simulink model "Robot2dof_control_Friction_RBFNN"  (Simulink 8.5)
settings: Solver=ode45  StartTime=0.0  StopTime=20  RelTol=1e-3
values from neighbouring files (symbols this model uses):
  l1 = 1    [Inv_Kinematic.m]    (also in Parameters.m)
  l2 = 0.5    [Inv_Kinematic.m]    (also in Parameters.m)
  m1 = 2    [Parameters.m]
  m2 = 1    [Parameters.m]
libraries: mblibv1 x13
(part 2 of 2)

== matlab function Computed Torque Controller/Computed Torque/Computed torque controller ==
  data: q1 input double; Torque1 output double; Torque2 output double; q2 input double; q1_dot input double; q2_dot input double; qd1 input double; qd2 input double; qd1_dot input double; qd2_dot input double; qd1_dotdot input double; qd2_dotdot input double
function [Torque1,Torque2] = ComputedTorqueController(q1,q2,q1_dot,q2_dot,qd1,qd2,qd1_dot,qd2_dot,qd1_dotdot,qd2_dotdot)
%% Adjust the inputs to apply the formulas
%   q2 is initially the complement angle of link 2 to link 1.
%   In order to apply the formulas, we need to determine the angle 
%   between link 2 and the x-axis to apply the dynamic model.
%   The same things go to qd2, qd2_dot, qd2_dotdot and q2_dot

qd2 = qd1 + qd2;
qd2_dot = qd1_dot + qd2_dot;
qd2_dotdot = qd1_dotdot + qd2_dotdot;
q2 = q1 + q2;
q2_dot = q1_dot + q2_dot;

%% Parameters
m1 = 2;
m2 = 1;
l1 = 1;
l2 = 0.5;
lc1 = .5;
lc2 = .25;

g = 9.81;
I1 = 4.3e-3;
I2 = 4.3e-3;

%% Compute dynamic model
M11 = m1*lc1^2 + m2*(l2^2+lc2^2+2*l1*lc2^2+2*l1*lc2*cos(q2))+I1+I2;
M12 = m2*(lc2^2+l1*lc2*cos(q2)) + I2;
M21 = M12;
M22 = m2*lc2^2 + I2;

M = [M11, M12; M21, M22];

h = -m2*l1*lc2*sin(q2);

C = [h*q2_dot, h*q2_dot+h*q1_dot;
     -h*q1_dot, 0];
 
G = [(m1*lc1+m2*l1)*g*cos(q1)+m2*lc2*g*cos(q1+q2);
     m2*lc2*g*cos(q1+q2)];
%% Computed torque controller
e1 = qd1 - q1;
e2 = qd2 - q2;
E = [e1; e2];

e1_dot = qd1_dot - q1_dot;
e2_dot = qd2_dot - q2_dot;
E_dot = [e1_dot; e2_dot];

Q_dot = [q1_dot; q2_dot];
Qd_dotdot = [qd1_dotdot; qd2_dotdot];

% kp1 = 1750;
% kp2 = 1300;
% 
%  kd1 = 46;
%  kd2 = 40;


% kp1 = 15000;
% kp2 = 16500;
% 
% kd1 = 360;
% kd2 = 600;

% kp1 = 1250;
% kp2 = 915;
% 
%  kd1 = 41;
%  kd2 = 31;

kp1 = 1550;
kp2 = 935;

 kd1 = 43;
 kd2 = 33;

Kp = [kp1, 0; 
      0, kp2];
  
Kd = [kd1, 0; 
      0, kd2];  

 
Torque = M*(Qd_dotdot + Kp*E + Kd*E_dot) + C*Q_dot + G;
 
Torque1 = Torque(1,1);
Torque2 = Torque(2,1);

== matlab function Computed Torque Controller/Neural Network /RBF for q2 ==
  data: Tnn2 output double; qa2 input double; qa2_dot input double; qda2 input double; qda2_dot input double
function Tnn2  = NeuralNetwork(qa2,qa2_dot,qda2,qda2_dot)
N=121;
M = sqrt(N);
persistent C X  var centerx centery CENTER_X CENTER_Y

%% Initialize the weighted matrices
if isempty(C)
    C = 0.1*ones(N,1);              % Output weight
    var = 0.141*ones(N,1);        % variance (sigma)
    centerx = -0.1:0.02:0.1;        % centers
    centery = -3:0.6:3;
    X = ones(2,1);                     % Input
    [CENTER_X,CENTER_Y] = meshgrid(centerx,centery);
end

%% Input of neural network

x1 = qa2 - qda2;                       % error
x2 = qa2_dot - qda2_dot;           % error_dot

X(1) = x1;
X(2) = x2;

  


%% Replaced function
% lamda1 = 0.005;
% s1 = (qa2 - qda2) + lamda1*(qa2_dot - qda2_dot);
lamda1 =  0.3;
lamda2 = 1;
% lamda1 = 1;
% lamda2 = 13;
s1 = (qa2 - qda2)*lamda2 + lamda1*(qa2_dot - qda2_dot);
S = s1;


%% HIDDEN LAYER (The basis function is chosen as Gaussian function)

R_temp = zeros(M,M);

for i = 1:10
    for j = 1:10
        R_temp(i,j) = (X(1)-CENTER_X(i,j))^2 + (X(2)-CENTER_Y(i,j))^2;
         R_temp(i,j) =  (R_temp(i,j)/(var(i*M-M+j)^2))/2;
          R_temp(i,j) = exp(-R_temp(i,j));
%R_temp(i,j) = exp(-(norm(X(1),CENTER_X(i,j))/var(i*5+j-5))^2/2)* exp(-(norm(X(2),CENTER_Y(i,j))/var(i*5+j-5))^2/2);
    end
end

% Create row(column) vector
k = 1;
Rx = zeros(1,N);
for i=1:M
    for j=1:M
    Rx(k) = R_temp(i,j);
    k= k+1;
    end
end

%% OUTPUT LAYER
T_net = zeros(1,1);
    for j=1:N
        T_net = T_net + C(j)*Rx(j);
    end



%% UPDATE WEIGHTS 
    % Learning rate
    m = 0.1; % weight learning rate
    n = 0.05; % center learning rate
    sg = 0.1; % sigma learing rate
  
% Update for ouput weights
for j = 1:N
    
       C(j) = C(j) - m*abs(S)*C(j) - m*S*Rx(j);
end

%Update for centers
% for j = 1:N
%     CENTER_X(j)  =  CENTER_X(j) - n*S*CENTER_X(j);
%     CENTER_Y(j)  =  CENTER_Y(j) - n*S*CENTER_Y(j);
% end
% 
% % Update for variance
% for j = 1:N
%     var(j) = var(j) - sg*S*var(j);
% end

Tnn2 = T_net;
end

== matlab function Mechanical Model. Two-link Arm/Coulomb & Viscous Friction/Embedded MATLAB Function ==
  data: u input double; y output double
function y = Sat(u)

if (abs(u)>0.01)
    y = sign(u);
else
    y = u/0.01;
end
